simulink model "ARDroneHover_AMOSTROU"  (R2017b)
settings: Solver=ode1  StartTime=0.0  StopTime=inf  FixedStep=sampleTime  RelTol=1e-3  EnableMultiTasking=on
values from neighbouring files (symbols this model uses):
  sampleTime = 1/200    (= 0.005)    [setupWPTracking.m]
undefined symbols (not defined in the file or in its folder): Standard_Devices, UDP_Protocol
libraries: sldrtlib x3, ARBlocks x2
(part 1 of 2)
CloseFcn:
  | rtwprivate ssgencode ModelCloseRequest Good_NL_model
settings Model: SimulationMode=external  ExtModeTrigDuration=100000  Creator=Paul  LastModifiedBy=PauloOliveira
settings DataIOCC: LimitDataPoints=on  SaveFormat=Array  SignalLoggingSaveFormat=ModelDataLogs  TimeSaveName=time
settings OptimizationCC: ExpressionDepthLimit=2147483647  InitFltsAndDblsToZero=on
settings DebuggingCC: UnderspecifiedInitializationDetection=Classic  MergeDetectMultiDrivingBlocksExec=none  SolverPrmCheckMsg=warning  FcnCallInpInsideContextMsg=warning  StateNameClashWarn=warning  SFUnexpectedBacktrackingDiag=warning  SFNoUnconditionalDefaultTransitionDiag=warning  SFExecutionAtInitializationDiag=none
settings HardwareCC: ProdBitPerLong=64  ProdHWDeviceType=Intel->x86-64 (Mac OS X)
settings ModelReferenceCC: PropagateSignalLabelsOutOfModel=off
settings RTWCC: SystemTargetFile=sldrt.tlc  TemplateMakefile=sldrt.tmf  Description=Simulink Desktop Real-Time  RTWCompilerOptimization=on
settings CodeAppCC: MaxIdLength=95  StateflowObjectComments=on
settings SimulinkDesktopRealTimeCC: TargetPreCompLibLocation=/Applications/MATLAB_R2017b.app/toolbox/sldrt/lib/maci64  TargetLangStandard=C89/C90 (ANSI)  SupportVariableSizeSignals=off
settings ConfigComp: CovMetricSettings=dw  CovHtmlReporting=on  CovSaveCumulativeToWorkspaceVar=on  CovSaveSingleToWorkspaceVar=on  CovExternalEMLEnable=off

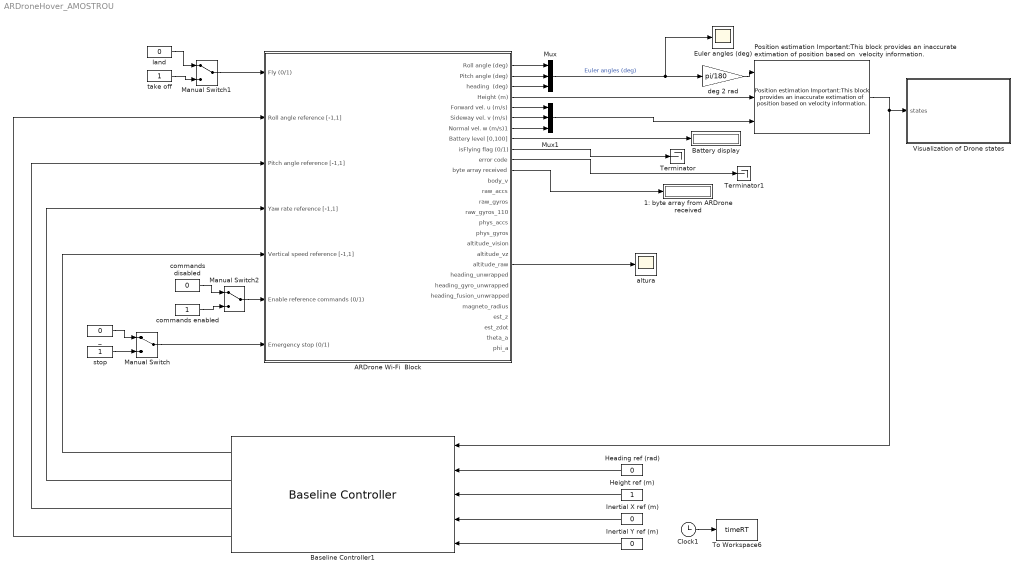
== system ARDroneHover_AMOSTROU ==
  "1: byte array from ARDrone received " : Display
  ARDrone Wi-Fi  Block : Subsystem  AncestorBlock="ARBlocks/ARDrone Wi-Fi  Block"
  Baseline Controller1 : ARBlocks/Baseline Controller
  Battery display : Display
  Clock1 : Clock
  Euler angles (deg) : Scope
  Heading ref (rad) : Constant  Value=0
  Height ref (m) : Constant
  Inertial X ref (m) : Constant  Value=0
  Inertial Y ref (m) : Constant  Value=0
  Manual Switch : ManualSwitch
  Manual Switch1 : ManualSwitch
  Manual Switch2 : ManualSwitch
  Mux : Mux  Inputs=3
  Mux1 : Mux  Inputs=3
  "Position estimation Important:This block provides an inaccurate extimation of position based on  velocity information. " : ARBlocks/Position estimation Important:This block provides an  inaccurate extimation of position  based on  velocity information. 
  Terminator : Terminator
  Terminator1 : Terminator
  To Workspace6 : ToWorkspace  VariableName=timeRT  SampleTime=sampleTime
  Visualization of Drone states : Subsystem
  _ : Constant  Value=0
  altura : Scope
  commands disabled : Constant  Value=0
  commands enabled : Constant
  deg 2 rad : Gain  Gain=pi/180
  land : Constant  Value=0
  stop : Constant
  take off : Constant
  wires:
  _/1 -> Manual Switch/1
  stop/1 -> Manual Switch/2
  land/1 -> Manual Switch1/1
  take off/1 -> Manual Switch1/2
  commands disabled/1 -> Manual Switch2/1
  commands enabled/1 -> Manual Switch2/2
  Manual Switch1/1 -> ARDrone Wi-Fi  Block/1(Fly (0/1))
  Manual Switch2/1 -> ARDrone Wi-Fi  Block/6(Enable reference commands (0/1))
  Manual Switch/1 -> ARDrone Wi-Fi  Block/7(Emergency stop (0/1))
  ARDrone Wi-Fi  Block/1(Roll angle (deg)) -> Mux/1
  ARDrone Wi-Fi  Block/2(Pitch angle (deg)) -> Mux/2
  ARDrone Wi-Fi  Block/5(Forward vel. u (m/s)) -> Mux1/1
  ARDrone Wi-Fi  Block/6(Sideway vel. v (m/s)) -> Mux1/2
  ARDrone Wi-Fi  Block/7(Normal vel. w (m/s)1) -> Mux1/3
  Mux/1 -> Euler angles (deg)/1, deg 2 rad/1  "Euler angles (deg)"
  ARDrone Wi-Fi  Block/8(Battery level [0,100]) -> Battery display/1
  Baseline Controller1/1 -> ARDrone Wi-Fi  Block/5(Vertical speed reference [-1,1])
  Baseline Controller1/3 -> ARDrone Wi-Fi  Block/3(Pitch angle reference [-1,1])
  "Position estimation Important:This block provides an inaccurate extimation of position based on  velocity information. "/1 -> Visualization of Drone states/1(states), Baseline Controller1/1
  deg 2 rad/1 -> "Position estimation Important:This block provides an inaccurate extimation of position based on  velocity information. "/1
  ARDrone Wi-Fi  Block/4(Height (m)) -> "Position estimation Important:This block provides an inaccurate extimation of position based on  velocity information. "/2
  Mux1/1 -> "Position estimation Important:This block provides an inaccurate extimation of position based on  velocity information. "/3
  Baseline Controller1/4 -> ARDrone Wi-Fi  Block/2(Roll angle reference [-1,1])
  ARDrone Wi-Fi  Block/3(heading  (deg)) -> Mux/3
  ARDrone Wi-Fi  Block/9(isFlying flag (0/1)) -> Terminator/1
  ARDrone Wi-Fi  Block/10(error code) -> Terminator1/1
  ARDrone Wi-Fi  Block/11(byte array received) -> "1: byte array from ARDrone received "/1
  Baseline Controller1/2 -> ARDrone Wi-Fi  Block/4(Yaw rate reference [-1,1])
  Clock1/1 -> To Workspace6/1
  Height ref (m)/1 -> Baseline Controller1/3
  Inertial X ref (m)/1 -> Baseline Controller1/4
  Inertial Y ref (m)/1 -> Baseline Controller1/5
  Heading ref (rad)/1 -> Baseline Controller1/2
  ARDrone Wi-Fi  Block/20(altitude_raw) -> altura/1

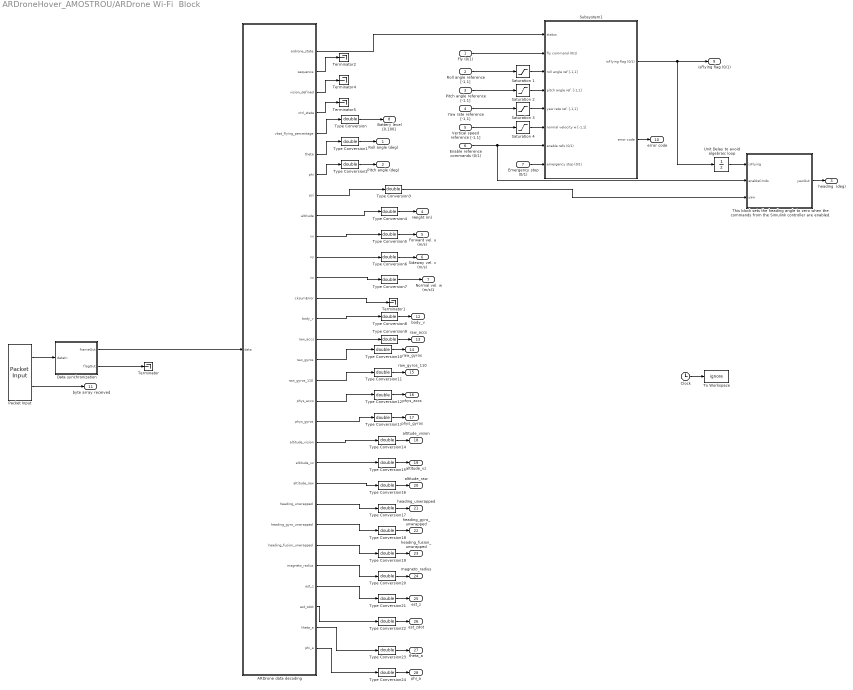
== system ARDroneHover_AMOSTROU/ARDrone Wi-Fi  Block ==
  Fly (0/1) : Inport
  Roll angle reference [-1,1] : Inport  Port=2
  Pitch angle reference [-1,1] : Inport  Port=3
  Yaw rate reference [-1,1] : Inport  Port=4
  Vertical speed reference [-1,1] : Inport  Port=5
  Enable reference commands (0/1) : Inport  Port=6
  Emergency stop (0/1) : Inport  Port=7
  ARDrone data decoding : MATLAB Function  TreatAsAtomicUnit=on
  Clock : Clock
      settings: Decimation=100
  "Data synchronization " : MATLAB Function  TreatAsAtomicUnit=on
  Packet Input : sldrtlib/Packet Input  SampleTime=sampleTime  MaxMissedTicks=100  ShowMissedTicks=off  YieldWhenWaiting=off  DrvName=Standard_Devices/UDP_Protocol  DrvAddress=5554  DrvOptions=[3232235777 5554]  PacketSize=2190  DataTypes='2190*uint8'  ShowReady=on  ShowError=off  PacketID=1  ByteOrder=1  ShowTimestamp=off
      settings: AttributesFormatString=UDP Protocol [5554]  SourceProductName=Simulink Desktop Real-Time
  Saturation {1..4} (4 alike) : Saturate  UpperLimit=1  LowerLimit=-1
  Subsystem1 : Subsystem
  Terminator{,1..2,4..5} (5 alike) : Terminator
  "This block sets the heading angle to zero when the commands from the Simulink controller are enabled. " : MATLAB Function  TreatAsAtomicUnit=on
  To Workspace : ToWorkspace  VariableName=ignore  SaveFormat=Timeseries  SampleTime=-1
  Type Conversion{,1..24} (25 alike) : DataTypeConversion  OutDataTypeStr=double
  Unit Delay to avoid algebraic loop : UnitDelay  SampleTime=-1
  Roll angle (deg) : Outport
  Pitch angle (deg) : Outport  Port=2
  heading  (deg) : Outport  Port=3
  Height (m) : Outport  Port=4
  Forward vel. u (m/s) : Outport  Port=5
  Sideway vel. v (m/s) : Outport  Port=6
  Normal vel. w (m/s)1 : Outport  Port=7
  Battery level [0,100] : Outport  Port=8
  isFlying flag (0/1) : Outport  Port=9
  error code : Outport  Port=10
  byte array received : Outport  Port=11
  body_v : Outport  Port=12
  raw_accs : Outport  Port=13
  raw_gyros : Outport  Port=14
  raw_gyros_110 : Outport  Port=15
  phys_accs : Outport  Port=16
  phys_gyros : Outport  Port=17
  altitude_vision : Outport  Port=18
  altitude_vz : Outport  Port=19
  altitude_raw : Outport  Port=20
  heading_unwrapped : Outport  Port=21
  heading_gyro_unwrapped : Outport  Port=22
  heading_fusion_unwrapped : Outport  Port=23
  magneto_radius : Outport  Port=24
  est_z : Outport  Port=25
  est_zdot : Outport  Port=26
  theta_a : Outport  Port=27
  phi_a : Outport  Port=28
  wires:
  Packet Input/1 -> "Data synchronization "/1(dataIn)
  "Data synchronization "/1(frameOut) -> ARDrone data decoding/1(data)
  Packet Input/2 -> byte array received/1
  ARDrone data decoding/1(ardrone_state) -> Subsystem1/1(status)
  Roll angle reference [-1,1]/1 -> Saturation 1/1
  Pitch angle reference [-1,1]/1 -> Saturation 2/1
  Yaw rate reference [-1,1]/1 -> Saturation 3/1
  Vertical speed reference [-1,1]/1 -> Saturation 4/1
  Enable reference commands (0/1)/1 -> "This block sets the heading angle to zero when the commands from the Simulink controller are enabled. "/2(enableCmds), Subsystem1/7(enable refs (0/1))
  Emergency stop (0/1)/1 -> Subsystem1/8(emergency stop (0/1))
  Subsystem1/1(isFlying flag (0/1)) -> isFlying flag (0/1)/1, Unit Delay to avoid algebraic loop/1
  Subsystem1/2(error code) -> error code/1
  ARDrone data decoding/13(cksumError) -> Terminator1/1
  Type Conversion/1 -> Battery level [0,100]/1
  Type Conversion1/1 -> Roll angle (deg)/1
  Type Conversion2/1 -> Pitch angle (deg)/1
  Type Conversion4/1 -> Height (m)/1
  Type Conversion5/1 -> Forward vel. u (m/s)/1
  Type Conversion6/1 -> Sideway vel. v (m/s)/1
  Type Conversion7/1 -> Normal vel. w (m/s)1/1
  Type Conversion3/1 -> "This block sets the heading angle to zero when the commands from the Simulink controller are enabled. "/3(yaw)
  "This block sets the heading angle to zero when the commands from the Simulink controller are enabled. "/1(yawOut) -> heading  (deg)/1
  Fly (0/1)/1 -> Subsystem1/2(fly command (0/1))
  Saturation 1/1 -> Subsystem1/3(roll angle ref [-1,1])
  Saturation 2/1 -> Subsystem1/4(pitch angle ref. [-1,1])
  Saturation 3/1 -> Subsystem1/5(yaw rate ref. [-1,1])
  Saturation 4/1 -> Subsystem1/6(normal velocity w [-1,1])
  "Data synchronization "/2(flagOut) -> Terminator/1
  Unit Delay to avoid algebraic loop/1 -> "This block sets the heading angle to zero when the commands from the Simulink controller are enabled. "/1(isFlying)
  Clock/1 -> To Workspace/1
  ARDrone data decoding/12(vz) -> Type Conversion7/1
  ARDrone data decoding/11(vy) -> Type Conversion6/1
  ARDrone data decoding/10(vx) -> Type Conversion5/1
  ARDrone data decoding/9(altitude) -> Type Conversion4/1
  ARDrone data decoding/8(psi) -> Type Conversion3/1
  ARDrone data decoding/7(phi) -> Type Conversion2/1
  ARDrone data decoding/6(theta) -> Type Conversion1/1
  ARDrone data decoding/5(vbat_flying_percentage) -> Type Conversion/1
  ARDrone data decoding/2(sequence) -> Terminator2/1
  ARDrone data decoding/3(vision_defined) -> Terminator4/1
  ARDrone data decoding/4(ctrl_state) -> Terminator5/1
  Type Conversion8/1 -> body_v/1
  Type Conversion9/1 -> raw_accs/1
  Type Conversion10/1 -> raw_gyros/1
  Type Conversion11/1 -> raw_gyros_110/1
  Type Conversion12/1 -> phys_accs/1
  Type Conversion13/1 -> phys_gyros/1
  ARDrone data decoding/19(phys_gyros) -> Type Conversion13/1
  Type Conversion14/1 -> altitude_vision/1
  Type Conversion15/1 -> altitude_vz/1
  Type Conversion16/1 -> altitude_raw/1
  Type Conversion17/1 -> heading_unwrapped/1
  Type Conversion18/1 -> heading_gyro_unwrapped/1
  Type Conversion19/1 -> heading_fusion_unwrapped/1
  Type Conversion20/1 -> magneto_radius/1
  Type Conversion21/1 -> est_z/1
  Type Conversion22/1 -> est_zdot/1
  ARDrone data decoding/28(est_zdot) -> Type Conversion22/1
  Type Conversion23/1 -> theta_a/1
  Type Conversion24/1 -> phi_a/1
  ARDrone data decoding/29(theta_a) -> Type Conversion23/1
  ARDrone data decoding/30(phi_a) -> Type Conversion24/1
  ARDrone data decoding/14(body_v) -> Type Conversion8/1
  ARDrone data decoding/15(raw_accs) -> Type Conversion9/1
  ARDrone data decoding/16(raw_gyros) -> Type Conversion10/1
  ARDrone data decoding/17(raw_gyros_110) -> Type Conversion11/1
  ARDrone data decoding/18(phys_accs) -> Type Conversion12/1
  ARDrone data decoding/20(altitude_vision) -> Type Conversion14/1
  ARDrone data decoding/21(altitude_vz) -> Type Conversion15/1
  ARDrone data decoding/22(altitude_raw) -> Type Conversion16/1
  ARDrone data decoding/23(heading_unwrapped) -> Type Conversion17/1
  ARDrone data decoding/24(heading_gyro_unwrapped) -> Type Conversion18/1
  ARDrone data decoding/25(heading_fusion_unwrapped) -> Type Conversion19/1
  ARDrone data decoding/26(magneto_radius) -> Type Conversion20/1
  ARDrone data decoding/27(est_z) -> Type Conversion21/1

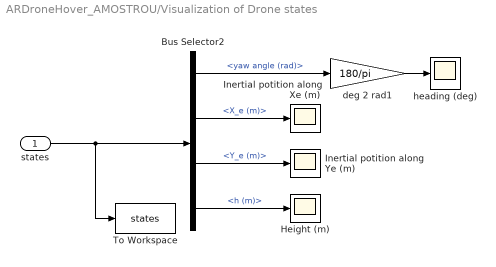
== system ARDroneHover_AMOSTROU/Visualization of Drone states ==
  states : Inport
  Bus Selector2 : BusSelector  OutputSignals=yaw angle (rad),X_e (m),Y_e (m),h (m)
  Height (m) : Scope
  Inertial potition along Xe (m) : Scope
  Inertial potition along Ye (m) : Scope
  To Workspace : ToWorkspace  VariableName=states  SaveFormat=Structure With Time  SampleTime=-1
  deg 2 rad1 : Gain  Gain=180/pi
  heading (deg) : Scope
  wires:
  states/1 -> To Workspace/1, Bus Selector2/1
  Bus Selector2/1 -> deg 2 rad1/1  "<yaw angle (rad)>"
  Bus Selector2/2 -> Inertial potition along Xe (m)/1  "<X_e (m)>"
  Bus Selector2/3 -> Inertial potition along Ye (m)/1  "<Y_e (m)>"
  Bus Selector2/4 -> Height (m)/1  "<h (m)>"
  deg 2 rad1/1 -> heading (deg)/1

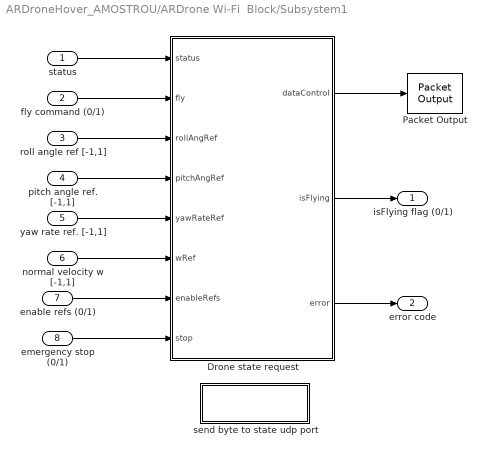
== system ARDroneHover_AMOSTROU/ARDrone Wi-Fi  Block/Subsystem1 ==
  status : Inport
  fly command (0/1) : Inport  Port=2
  roll angle ref [-1,1] : Inport  Port=3
  pitch angle ref. [-1,1] : Inport  Port=4
  yaw rate ref. [-1,1] : Inport  Port=5
  normal velocity w [-1,1] : Inport  Port=6
  enable refs (0/1) : Inport  Port=7
  emergency stop (0/1) : Inport  Port=8
  Drone state request : MATLAB Function  TreatAsAtomicUnit=on  SystemSampleTime=sampleTime
  Packet Output : sldrtlib/Packet Output  SampleTime=-1  MaxMissedTicks=100  ShowMissedTicks=off  YieldWhenWaiting=off  DrvName=Standard_Devices/UDP_Protocol  DrvAddress=5556  DrvOptions=[3232235777 5556]  PacketSize=150  DataTypes='150*uint8'  ShowReady=off  ShowError=off  PacketID=1  ByteOrder=1  InitialValue=[]  FinalValue=[]
      settings: AttributesFormatString=UDP Protocol [5556]  SourceProductName=Simulink Desktop Real-Time
  "send byte to state udp port " : Subsystem
  isFlying flag (0/1) : Outport
  error code : Outport  Port=2
  wires:
  fly command (0/1)/1 -> Drone state request/2(fly)
  pitch angle ref. [-1,1]/1 -> Drone state request/4(pitchAngRef)
  status/1 -> Drone state request/1(status)
  Drone state request/1(dataControl) -> Packet Output/1
  Drone state request/2(isFlying) -> isFlying flag (0/1)/1
  roll angle ref [-1,1]/1 -> Drone state request/3(rollAngRef)
  yaw rate ref. [-1,1]/1 -> Drone state request/5(yawRateRef)
  normal velocity w [-1,1]/1 -> Drone state request/6(wRef)
  enable refs (0/1)/1 -> Drone state request/7(enableRefs)
  emergency stop (0/1)/1 -> Drone state request/8(stop)
  Drone state request/3(error) -> error code/1

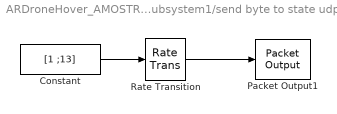
== system ARDroneHover_AMOSTROU/ARDrone Wi-Fi  Block/Subsystem1/send byte to state udp port  ==
  Constant : Constant  Value=[1 ;13]  OutDataTypeStr=uint8
  Packet Output1 : sldrtlib/Packet Output  SampleTime=sampleTime*10  MaxMissedTicks=100  ShowMissedTicks=off  YieldWhenWaiting=off  DrvName=Standard_Devices/UDP_Protocol  DrvAddress=5554  DrvOptions=[3232235777 5554]  PacketSize=2  DataTypes='2*uint8'  ShowReady=off  ShowError=off  PacketID=1  ByteOrder=1  InitialValue=[]  FinalValue=[]
      settings: AttributesFormatString=UDP Protocol [5554]  SourceProductName=Simulink Desktop Real-Time
  Rate Transition : RateTransition  OutPortSampleTime=sampleTime*10
  wires:
  Constant/1 -> Rate Transition/1
  Rate Transition/1 -> Packet Output1/1

== matlab function ARDroneHover_AMOSTROU/ARDrone Wi-Fi  Block/ARDrone data decoding ==
  data: ardrone_state output; sequence output; vision_defined output; data input; ctrl_state output; vbat_flying_percentage output; theta output; phi output; psi output; altitude output; vx output; vy output; vz output; cksumError output; body_v output; raw_accs output; raw_gyros output; raw_gyros_110 output; phys_accs output; phys_gyros output; altitude_vision output; altitude_vz output; altitude_raw output; heading_unwrapped output; heading_gyro_unwrapped output; heading_fusion_unwrapped output; magneto_radius output; est_z output; est_zdot output; theta_a output; phi_a output
function [ ardrone_state, sequence, vision_defined, ctrl_state, vbat_flying_percentage, theta, phi, psi, altitude, vx, vy, vz , cksumError , body_v,raw_accs,raw_gyros,raw_gyros_110,phys_accs,phys_gyros,altitude_vision,altitude_vz,altitude_raw,heading_unwrapped,heading_gyro_unwrapped,heading_fusion_unwrapped,magneto_radius,est_z,est_zdot,theta_a,phi_a]= fcn(data)
%#codegen

%initialie arrays
raw_accs=zeros(3,1);
raw_gyros=zeros(3,1);
raw_gyros_110=zeros(2,1);
phys_accs=zeros(3,1);
phys_gyros=zeros(3,1);
offsets_g=zeros(3,1);
obs_x=zeros(3,1);
est_vb=zeros(2,1);
of_dx=zeros(5,1);
of_dy=zeros(5,1);
body_v=zeros(3,1);
time_custom=zeros(20,1);
locked=zeros(30,1);
point=zeros(30,2);
type=zeros(4,1);
xc=zeros(4,1);
yc=zeros(4,1);
width=zeros(4,1);
height=zeros(4,1);
dist=zeros(4,1);
orientation_angle=zeros(4,1);
rotation=zeros(3,3,4);
translation=zeros(3,1,4);
camera_source=zeros(4,1);
data_frame=zeros(32,1);
magneto_raw=zeros(3,1);
magneto_rectified=zeros(3,1);
magneto_offset=zeros(3,1);

% Checksum array. cksum(1) contains the computed checksum, cksum(2)
% contains the checksum sent by the ARDrone. 
cksum = [0 0 ]; 

% Previous value of height 
persistent hPrev ; 
% Previous data packet
persistent dataPrev ; 

% Initialization of persistent variables
if isempty(hPrev)
    hPrev=0 ; 
end

if isempty(dataPrev)
    dataPrev = uint8(zeros(2186,1)) ;
end

% Computing checksum
cksum(1) =  sum(double(data(1:end-8))) +442; 
% Checksum given by the drone
cksum(2) = double(data(end-3)) + double(data(end-2))*256 +  double(data(end-1))*256^2 + double(data(end))*256^3 ; 
% Checksum error
cksumError = abs(cksum(1)-cksum(2));
%% Change the following if statement to ensure that the data checksum is valid 
%if (data(15) == 148 && cksumError==0 )
if (data(15) == 148  )
    dataPrev = data; 
else
    data = dataPrev; 
end

% Converting bytes to drone information

% header data
ardrone_state = getDroneState(data(1:4));
sequence = decode_32bit(data(5:8),1);
vision_defined = data(9);

% demo data
ctrl_state = decode_32bit(data(17:20),1);
vbat_flying_percentage = decode_32bit(data(21:24),1); % unit: deg
theta = decode_32bit(data(25:28),0)/1000; % unit: deg
phi = decode_32bit(data(29:32),0)/1000; % unit: deg
psi = decode_32bit(data(33:36),0)/1000; % unit: deg
altitude = decode_32bit(data(37:40),1)/1000; % unit: deg
vx = decode_32bit(data(41:44),0)/1000; % unit: m/s
vy = decode_32bit(data(45:48),0)/1000; % unit: m/s
vz = decode_32bit(data(49:52),0)/1000; % unit: m/s
detection_camera_type = decode_32bit(data(109:112),1);

%altitude = decode_32bit(data(113:116),1)/1000;

% time !!!!CHECK UNITS!!!!
time = decode_32bit(data(165:168),1);

% raw data
raw_accs(1) = decode_16bit(data(173:174),0);
raw_accs(2) = decode_16bit(data(175:176),0);
raw_accs(3) = decode_16bit(data(177:178),0);
raw_gyros(1) = decode_16bit(data(179:180),1);
raw_gyros(2) = decode_16bit(data(181:182),1);
raw_gyros(3) = decode_16bit(data(183:184),1);
raw_gyros_110(1) = decode_16bit(data(185:186),1);
raw_gyros_110(2) = decode_16bit(data(187:188),1);
vbat_raw = decode_32bit(data(189:192),0);
us_debut_echo = decode_16bit(data(193:194),0);
us_fin_echo = decode_16bit(data(195:196),0);
us_association_echo = decode_16bit(data(197:198),0);
us_distance_echo = decode_16bit(data(199:200),0);
us_courbe_temps = decode_16bit(data(201:202),0);
us_courbe_valeur = decode_16bit(data(203:204),0);
us_courbe_ref = decode_16bit(data(205:206),0);
flag_echo_ini = decode_16bit(data(207:208),0);
nb_echo = decode_16bit(data(209:210),0);
sum_echo = decode_32bit(data(211:214),1);
alt_temp_raw = decode_32bit(data(215:218),2);
gradient = decode_16bit(data(219:220),1);

% physycal measures
accs_temp = decode_32bit(data(225:228),0);
gyro_temp = decode_16bit(data(229:230),0);
phys_accs(1) = decode_32bit(data(231:234),0);
phys_accs(2) = decode_32bit(data(235:238),0);
phys_accs(3) = decode_32bit(data(239:242),0);
phys_gyros(1) = decode_32bit(data(243:246),0);
phys_gyros(2) = decode_32bit(data(247:250),0);
phys_gyros(3) = decode_32bit(data(251:254),0);
alim3V3 = decode_32bit(data(255:258),1);
vrefEpson = decode_32bit(data(259:262),1);
vrefIDG = decode_32bit(data(263:266),1);

% gyros offsets
offsets_g(1) = decode_32bit(data(271:274),0);
offsets_g(2) = decode_32bit(data(275:278),0);
offsets_g(3) = decode_32bit(data(279:282),0);

% euler angles
theta_a = decode_32bit(data(287:290),0);
phi_a = decode_32bit(data(291:294),0);

% referenes
ref_theta = decode_32bit(data(299:302),2);
ref_phi = decode_32bit(data(303:306),2);
ref_theta_I = decode_32bit(data(307:310),2);
ref_phi_I = decode_32bit(data(311:314),2);
ref_pitch = decode_32bit(data(315:318),2);
ref_roll = decode_32bit(data(319:322),2);
ref_yaw = decode_32bit(data(323:326),2);
ref_psi = decode_32bit(data(327:330),2);
vx_ref = decode_32bit(data(331:334),0);
vy_ref = decode_32bit(data(335:338),0);
theta_mod = decode_32bit(data(339:342),0);
phi_mod = decode_32bit(data(343:346),0);
k_v_x = decode_32bit(data(347:350),0);
k_v_y = decode_32bit(data(351:354),0);
k_mode = decode_32bit(data(355:358),1);
ui_time = decode_32bit(data(359:362),0);
ui_theta = decode_32bit(data(363:366),0);
ui_phi = decode_32bit(data(367:370),0);
ui_psi = decode_32bit(data(371:374),0);
ui_psi_accuracy = decode_32bit(data(375:378),0);
ui_seq = decode_32bit(data(379:382),2);

% trims
angular_rates_trim_r = decode_32bit(data(387:390),0);
euler_angles_trim_theta = decode_32bit(data(391:394),0);
euler_angles_trim_phi = decode_32bit(data(395:398),0);

% rc_refereces
rc_ref_pitch = decode_32bit(data(403:406),2);
rc_ref_roll = decode_32bit(data(407:410),2);
rc_ref_yaw = decode_32bit(data(411:414),2);
rc_ref_gaz = decode_32bit(data(415:418),2);
rc_ref_ag = decode_32bit(data(419:422),2);

% pwm
motor1 = data(427);
motor2 = data(428);
motor3 = data(429);
motor4 = data(430);
sat_motor1 = data(431);
sat_motor2 = data(432);
sat_motor3 = data(433);
sat_motor4 = data(434);
gaz_feed_forward = decode_32bit(data(435:438),0);
gaz_altitude = decode_32bit(data(439:442),0);
altitude_integral = decode_32bit(data(443:446),0);
vz_ref = decode_32bit(data(447:450),0);
u_pitch = decode_32bit(data(451:454),2);
u_roll = decode_32bit(data(455:458),2);
u_yaw = decode_32bit(data(459:462),2);
yaw_u_I = decode_32bit(data(463:466),0);
u_pitch_planif = decode_32bit(data(467:470),2);
u_roll_planif = decode_32bit(data(471:474),2);
u_yaw_planif = decode_32bit(data(475:478),2);
u_gaz_planif = decode_32bit(data(479:482),0);
current_motor1 = decode_16bit(data(483:484),0);
current_motor2 = decode_16bit(data(485:486),0);
current_motor3 = decode_16bit(data(487:488),0);
current_motor4 = decode_16bit(data(489:490),0);
altitude_prop = decode_32bit(data(491:494),0);
altitude_der = decode_32bit(data(495:498),0);

% altitude
altitude_vision = decode_32bit(data(519:522),2);
altitude_vz = decode_32bit(data(523:526),0);
altitude_ref = decode_32bit(data(527:530),2);
altitude_raw = decode_32bit(data(531:534),2);
obs_accZ = decode_32bit(data(535:538),0);
obs_alt = decode_32bit(data(539:542),0);
obs_x(1) = decode_32bit(data(543:546),0);
obs_x(2) = decode_32bit(data(547:550),0);
obs_x(3) = decode_32bit(data(551:554),0);
obs_state = decode_32bit(data(555:558),1);
est_vb(1) = decode_32bit(data(559:562),0);
est_vb(2) = decode_32bit(data(563:566),0);
est_state = decode_32bit(data(567:570),1);

% vision_raw
vision_tx_raw = decode_32bit(data(575:578),0);
vision_ty_raw = decode_32bit(data(579:582),0);
vision_tz_raw = decode_32bit(data(583:586),0);

% vision_of
of_dx(1) = decode_32bit(data(591:594),0);
of_dx(2) = decode_32bit(data(595:598),0);
of_dx(3) = decode_32bit(data(599:602),0);
of_dx(4) = decode_32bit(data(603:606),0);
of_dx(5) = decode_32bit(data(607:610),0);
of_dy(1) = decode_32bit(data(611:614),0);
of_dy(2) = decode_32bit(data(615:618),0);
of_dy(3) = decode_32bit(data(619:622),0);
of_dy(4) = decode_32bit(data(623:626),0);
of_dy(5) = decode_32bit(data(627:630),0);

% vision
vision_state = decode_32bit(data(635:638),1);
vision_misc = decode_32bit(data(639:642),2);
vision_phi_trim = decode_32bit(data(643:646),0);
vision_phi_ref_prop = decode_32bit(data(647:650),0);
vision_theta_trim = decode_32bit(data(651:654),0);
vision_theta_ref_prop = decode_32bit(data(655:658),0);
new_raw_picture = decode_32bit(data(659:662),2);
theta_capture = decode_32bit(data(663:666),0);
phi_capture = decode_32bit(data(667:670),0);
psi_capture = decode_32bit(data(671:674),0);
altitude_capture = decode_32bit(data(675:678),2);
time_capture = decode_32bit(data(679:682),1);
body_v(1) = decode_32bit(data(683:686),0);
body_v(2) = decode_32bit(data(687:690),0);
body_v(3) = decode_32bit(data(691:694),0);
delta_phi = decode_32bit(data(695:698),0);
delta_theta = decode_32bit(data(699:702),0);
delta_psi = decode_32bit(data(703:706),0);
gold_defined = decode_32bit(data(707:710),1);
gold_reset = decode_32bit(data(711:714),1);
gold_x = decode_32bit(data(715:718),0);
gold_y = decode_32bit(data(719:722),0);

% vision perf
time_szo = decode_32bit(data(727:730),0);
time_corners = decode_32bit(data(731:734),0);
time_compute = decode_32bit(data(725:738),0);
time_tracking = decode_32bit(data(739:742),0);
time_trans = decode_32bit(data(743:746),0);
time_update = decode_32bit(data(747:750),0);
time_custom(1) = decode_32bit(data(751:754),0);
time_custom(2) = decode_32bit(data(755:758),0);
time_custom(3) = decode_32bit(data(759:762),0);
time_custom(4) = decode_32bit(data(763:766),0);
time_custom(5) = decode_32bit(data(767:770),0);
time_custom(6) = decode_32bit(data(771:774),0);
time_custom(7) = decode_32bit(data(775:778),0);
time_custom(8) = decode_32bit(data(779:782),0);
time_custom(9) = decode_32bit(data(783:786),0);
time_custom(10) = decode_32bit(data(787:790),0);
time_custom(11) = decode_32bit(data(791:794),0);
time_custom(12) = decode_32bit(data(795:798),0);
time_custom(13) = decode_32bit(data(799:802),0);
time_custom(14) = decode_32bit(data(803:806),0);
time_custom(15) = decode_32bit(data(807:810),0);
time_custom(16) = decode_32bit(data(811:814),0);
time_custom(17) = decode_32bit(data(815:818),0);
time_custom(18) = decode_32bit(data(819:822),0);
time_custom(19) = decode_32bit(data(823:826),0);
time_custom(20) = decode_32bit(data(827:830),0);

% trackers send
locked(1) = decode_32bit(data(835:838),2);
locked(2) = decode_32bit(data(839:842),2);
locked(3) = decode_32bit(data(843:846),2);
locked(4) = decode_32bit(data(847:850),2);
locked(5) = decode_32bit(data(851:854),2);
locked(6) = decode_32bit(data(855:858),2);
locked(7) = decode_32bit(data(859:862),2);
locked(8) = decode_32bit(data(863:866),2);
locked(9) = decode_32bit(data(867:870),2);
locked(10) = decode_32bit(data(871:874),2);
locked(11) = decode_32bit(data(875:878),2);
locked(12) = decode_32bit(data(879:882),2);
locked(13) = decode_32bit(data(883:886),2);
locked(14) = decode_32bit(data(887:890),2);
locked(15) = decode_32bit(data(891:894),2);
locked(16) = decode_32bit(data(895:898),2);
locked(17) = decode_32bit(data(899:902),2);
locked(18) = decode_32bit(data(903:906),2);
locked(19) = decode_32bit(data(907:910),2);
locked(20) = decode_32bit(data(911:914),2);
locked(21) = decode_32bit(data(915:918),2);
locked(22) = decode_32bit(data(919:922),2);
locked(23) = decode_32bit(data(923:926),2);
locked(24) = decode_32bit(data(927:930),2);
locked(25) = decode_32bit(data(931:934),2);
locked(26) = decode_32bit(data(935:938),2);
locked(27) = decode_32bit(data(939:942),2);
locked(28) = decode_32bit(data(943:946),2);
locked(29) = decode_32bit(data(947:950),2);
locked(30) = decode_32bit(data(951:954),2);
point(1,1) = decode_32bit(data(955:958),0);
point(1,2) = decode_32bit(data(959:962),0);
point(2,1) = decode_32bit(data(963:966),0);
point(2,2) = decode_32bit(data(967:970),0);
point(3,1) = decode_32bit(data(971:974),0);
point(3,2) = decode_32bit(data(975:978),0);
point(4,1) = decode_32bit(data(979:982),0);
point(4,2) = decode_32bit(data(983:986),0);
point(5,1) = decode_32bit(data(987:990),0);
point(5,2) = decode_32bit(data(991:994),0);
point(6,1) = decode_32bit(data(995:998),0);
point(6,2) = decode_32bit(data(999:1002),0);
point(7,1) = decode_32bit(data(1003:1006),0);
point(7,2) = decode_32bit(data(1007:1010),0);
point(8,1) = decode_32bit(data(1011:1014),0);
point(8,2) = decode_32bit(data(1015:1018),0);
point(9,1) = decode_32bit(data(1019:1022),0);
point(9,2) = decode_32bit(data(1023:1026),0);
point(10,1) = decode_32bit(data(1027:1030),0);
point(10,2) = decode_32bit(data(1031:1034),0);
point(11,1) = decode_32bit(data(1035:1038),0);
point(11,2) = decode_32bit(data(1039:1042),0);
point(12,1) = decode_32bit(data(1043:1046),0);
point(12,2) = decode_32bit(data(1047:1050),0);
point(13,1) = decode_32bit(data(1051:1054),0);
point(13,2) = decode_32bit(data(1055:1058),0);
point(14,1) = decode_32bit(data(1059:1062),0);
point(14,2) = decode_32bit(data(1063:1066),0);
point(15,1) = decode_32bit(data(1067:1070),0);
point(15,2) = decode_32bit(data(1071:1074),0);
point(16,1) = decode_32bit(data(1075:1078),0);
point(16,2) = decode_32bit(data(1079:1082),0);
point(17,1) = decode_32bit(data(1083:1086),0);
point(17,2) = decode_32bit(data(1087:1090),0);
point(18,1) = decode_32bit(data(1091:1094),0);
point(18,2) = decode_32bit(data(1095:1098),0);
point(19,1) = decode_32bit(data(1099:1102),0);
point(19,2) = decode_32bit(data(1103:1106),0);
point(20,1) = decode_32bit(data(1107:1110),0);
point(20,2) = decode_32bit(data(1111:1114),0);
point(21,1) = decode_32bit(data(1115:1118),0);
point(21,2) = decode_32bit(data(1119:1122),0);
point(22,1) = decode_32bit(data(1123:1126),0);
point(22,2) = decode_32bit(data(1127:1130),0);
point(23,1) = decode_32bit(data(1131:1134),0);
point(23,2) = decode_32bit(data(1135:1138),0);
point(24,1) = decode_32bit(data(1139:1142),0);
point(24,2) = decode_32bit(data(1143:1146),0);
point(25,1) = decode_32bit(data(1147:1150),0);
point(25,2) = decode_32bit(data(1151:1154),0);
point(26,1) = decode_32bit(data(1155:1158),0);
point(26,2) = decode_32bit(data(1159:1162),0);
point(27,1) = decode_32bit(data(1163:1166),0);
point(27,2) = decode_32bit(data(1167:1170),0);
point(28,1) = decode_32bit(data(1171:1174),0);
point(28,2) = decode_32bit(data(1175:1178),0);
point(29,1) = decode_32bit(data(1179:1182),0);
point(29,2) = decode_32bit(data(1183:1186),0);
point(30,1) = decode_32bit(data(1187:1190),0);
point(30,2) = decode_32bit(data(1191:1194),0);

% vision detect
nb_detected = decode_32bit(data(1199:1202),1);
type(1) = decode_32bit(data(1203:1206),1);
type(2) = decode_32bit(data(1207:1210),1);
type(3) = decode_32bit(data(1211:1214),1);
type(4) = decode_32bit(data(1215:1218),1);
xc(1) = decode_32bit(data(1219:1222),1);
xc(2) = decode_32bit(data(1223:1226),1);
xc(3) = decode_32bit(data(1227:1230),1);
xc(4) = decode_32bit(data(1231:1234),1);
yc(1) = decode_32bit(data(1235:1238),1);
yc(2) = decode_32bit(data(1239:1242),1);
yc(3) = decode_32bit(data(1243:1246),1);
yc(4) = decode_32bit(data(1247:1250),1);
width(1) = decode_32bit(data(1251:1254),1);
width(2) = decode_32bit(data(1255:1258),1);
width(3) = decode_32bit(data(1259:1262),1);
width(4) = decode_32bit(data(1263:1266),1);
height(1) = decode_32bit(data(1267:1270),1);
height(2) = decode_32bit(data(1271:1274),1);
height(3) = decode_32bit(data(1275:1278),1);
height(4) = decode_32bit(data(1279:1282),1);
dist(1) = decode_32bit(data(1283:1286),1);
dist(2) = decode_32bit(data(1287:1290),1);
dist(3) = decode_32bit(data(1291:1294),1);
dist(4) = decode_32bit(data(1295:1298),1);
orientation_angle(1) = decode_32bit(data(1299:1302),0);
orientation_angle(2) = decode_32bit(data(1303:1306),0);
orientation_angle(3) = decode_32bit(data(1307:1310),0);
orientation_angle(4) = decode_32bit(data(131:1314),0);
rotation(1,1,1) = decode_32bit(data(1315:1318),0);
rotation(1,2,1) = decode_32bit(data(1319:1322),0);
rotation(1,3,1) = decode_32bit(data(1323:1326),0);
rotation(2,1,1) = decode_32bit(data(1327:1330),0);
rotation(2,2,1) = decode_32bit(data(1331:1334),0);
rotation(2,3,1) = decode_32bit(data(1335:1338),0);
rotation(3,1,1) = decode_32bit(data(1339:1342),0);
rotation(3,2,1) = decode_32bit(data(1343:1346),0);
rotation(3,3,1) = decode_32bit(data(1347:1350),0);
rotation(1,1,2) = decode_32bit(data(1351:1354),0);
rotation(1,2,2) = decode_32bit(data(1355:1358),0);
rotation(1,3,2) = decode_32bit(data(1359:1362),0);
rotation(2,1,2) = decode_32bit(data(1363:1366),0);
rotation(2,2,2) = decode_32bit(data(1367:1370),0);
rotation(2,3,2) = decode_32bit(data(1371:1374),0);
rotation(3,1,2) = decode_32bit(data(1375:1378),0);
rotation(3,2,2) = decode_32bit(data(1379:1382),0);
rotation(3,3,2) = decode_32bit(data(1383:1386),0);
rotation(1,1,3) = decode_32bit(data(1387:1390),0);
rotation(1,2,3) = decode_32bit(data(1391:1394),0);
rotation(1,3,3) = decode_32bit(data(1395:1398),0);
rotation(2,1,3) = decode_32bit(data(1399:1402),0);
rotation(2,2,3) = decode_32bit(data(1403:1406),0);
rotation(2,3,3) = decode_32bit(data(1407:1410),0);
rotation(3,1,3) = decode_32bit(data(1411:1414),0);
rotation(3,2,3) = decode_32bit(data(1415:1418),0);
rotation(3,3,3) = decode_32bit(data(1419:1422),0);
rotation(1,1,4) = decode_32bit(data(1423:1426),0);
rotation(1,2,4) = decode_32bit(data(1427:1430),0);
rotation(1,3,4) = decode_32bit(data(1431:1434),0);
rotation(2,1,4) = decode_32bit(data(1435:1438),0);
rotation(2,2,4) = decode_32bit(data(1439:1442),0);
rotation(2,3,4) = decode_32bit(data(1443:1446),0);
rotation(3,1,4) = decode_32bit(data(1447:1450),0);
rotation(3,2,4) = decode_32bit(data(1451:1454),0);
rotation(3,3,4) = decode_32bit(data(1455:1458),0);
translation(1,1,1) = decode_32bit(data(1459:1462),0);
translation(1,1,1) = decode_32bit(data(1463:1466),0);
translation(3,1,1) = decode_32bit(data(1467:1470),0);
translation(1,1,2) = decode_32bit(data(1471:1474),0);
translation(2,1,2) = decode_32bit(data(1475:1478),0);
translation(3,1,2) = decode_32bit(data(1479:1482),0);
translation(1,1,3) = decode_32bit(data(1483:1486),0);
translation(2,1,3) = decode_32bit(data(1487:1490),0);
translation(3,1,3) = decode_32bit(data(1491:1494),0);
translation(1,1,4) = decode_32bit(data(1495:1498),0);
translation(2,1,4) = decode_32bit(data(1499:1502),0);
translation(3,1,4) = decode_32bit(data(1503:1506),0);
camera_source(1) = decode_32bit(data(1507:1510),1);
camera_source(2) = decode_32bit(data(1511:1514),1);
camera_source(3) = decode_32bit(data(1515:1518),1);
camera_source(4) = decode_32bit(data(1519:1522),1);

% watchdog
watchdog = decode_32bit(data(1527:1530),2);

% adc data frame
version = decode_32bit(data(1535:1538),1);
data_frame(1) = data(1539);
data_frame(2) = data(1540);
data_frame(3) = data(1541);
data_frame(4) = data(1542);
data_frame(5) = data(1543);
data_frame(6) = data(1544);
data_frame(7) = data(1545);
data_frame(8) = data(1546);
data_frame(9) = data(1547);
data_frame(10) = data(1548);
data_frame(11) = data(1549);
data_frame(12) = data(1550);
data_frame(13) = data(1551);
data_frame(14) = data(1552);
data_frame(15) = data(1553);
data_frame(16) = data(1554);
data_frame(17) = data(1555);
data_frame(18) = data(1556);
data_frame(19) = data(1557);
data_frame(20) = data(1558);
data_frame(21) = data(1559);
data_frame(22) = data(1560);
data_frame(23) = data(1561);
data_frame(24) = data(1562);
data_frame(25) = data(1563);
data_frame(26) = data(1564);
data_frame(27) = data(1565);
data_frame(28) = data(1566);
data_frame(29) = data(1567);
data_frame(30) = data(1568);
data_frame(31) = data(1569);
data_frame(32) = data(1570);

% video stream
quant = data(1575);
frame_size = decode_32bit(data(1576:1579),1);
frame_number = decode_32bit(data(1580:1583),1);
atcmd_ref_seq = decode_32bit(data(1584:1587),1);
atcmd_mean_ref_gap = decode_32bit(data(1588:1591),1);
atcmd_var_ref_gap = decode_32bit(data(1592:1595),0);
atcmd_ref_quality = decode_32bit(data(1596:1599),1);
out_bitrate = decode_32bit(data(1600:1603),1);
desired_bitrate = decode_32bit(data(1604:1607),1);
data1 = decode_32bit(data(1608:1611),2);
data2 = decode_32bit(data(1612:1615),2);
data3 = decode_32bit(data(1616:1619),2);
data4 = decode_32bit(data(1620:1623),2);
data5 = decode_32bit(data(1624:1627),2);
tcp_queue_level = decode_32bit(data(1628:1631),1);
fifo_queue_level = decode_32bit(data(1632:1635),1);

% games
double_tap_counter = decode_32bit(data(1640:1643),1);
finish_line_counter = decode_32bit(data(1644:1647),1);

% pressure_raw
up = decode_32bit(data(1652:1655),2);
ut = decode_16bit(data(1656:1657),1);
Temperature_meas = decode_32bit(data(1658:1661),2);
Precission_meas = decode_32bit(data(1662:1665),2);

% magneto
mx = decode_16bit(data(1670:1671),1);
my = decode_16bit(data(1672:1673),1);
mz = decode_16bit(data(1674:1675),1);
magneto_raw(1) = decode_32bit(data(1676:1679),0);
magneto_raw(2) = decode_32bit(data(1680:1683),0);
magneto_raw(3) = decode_32bit(data(1684:1687),0);
magneto_rectified(1) = decode_32bit(data(1688:1691),0);
magneto_rectified(2) = decode_32bit(data(1692:1695),0);
magneto_rectified(3) = decode_32bit(data(1696:1699),0);
magneto_offset(1) = decode_32bit(data(1700:1703),0);
magneto_offset(2) = decode_32bit(data(1704:1707),0);
magneto_offset(3) = decode_32bit(data(1708:1711),0);
heading_unwrapped = decode_32bit(data(1712:1715),0);
heading_gyro_unwrapped = decode_32bit(data(1716:1719),0);
heading_fusion_unwrapped = decode_32bit(data(1720:1723),0);
magneto_calibration_ok = char(data(1724:1732));
magneto_state = decode_32bit(data(1733:1736),1);
magneto_radius = decode_32bit(data(1737:1740),0);
error_mean = decode_32bit(data(1741:1744),0);
error_var = decode_32bit(data(1745:1748),0);

% wind speed
wind_speed = decode_32bit(data(1753:1756),0);
wind_angle = decode_32bit(data(1757:1760),0);
wind_compensation_theta = decode_32bit(data(1761:1764),0);
wind_compensation_phi = decode_32bit(data(1765:1768),0);
state_x1 = decode_32bit(data(1769:1772),0);
state_x2 = decode_32bit(data(1773:1776),0);
state_x3 = decode_32bit(data(1777:1780),0);
state_x4 = decode_32bit(data(1781:1784),0);
state_x5 = decode_32bit(data(1785:1788),0);
state_x6 = decode_32bit(data(1789:1792),0);
magneto_debug1 = decode_32bit(data(1793:1796),0);
magneto_debug2 = decode_32bit(data(1797:1800),0);
magneto_debug3 = decode_32bit(data(1801:1804),0);
% 8 bytes unacounted for!!

% kalman pressure
offset_pressure = decode_32bit(data(1817:1820),0);
est_z = decode_32bit(data(1821:1824),0);
est_zdot = decode_32bit(data(1825:1828),0);
est_bias_PWM = decode_32bit(data(1829:1832),0);
est_biais_pression = decode_32bit(data(1833:1836),0);
offset_US = decode_32bit(data(1837:1840),0);
prediction_US = decode_32bit(data(1841:1844),0);
cov_alt = decode_32bit(data(1817:1848),0);
cov_PWM = decode_32bit(data(1849:1852),0);
cov_vitesse = decode_32bit(data(1853:1856),0);
bool_effect_sol = data(1857);
somme_inno = decode_32bit(data(1861:1864),0);
flag_reject_US = data(1865);
u_multisinus = decode_32bit(data(1869:1872),0);
gaz_altitude = decode_32bit(data(1873:1876),0);
Flag_multissinus = data(1877);
Flag_multissinus_debut = data(1881);

% hdvideo stream
hdvideo_state = decode_32bit(data(1889:1892),1);
storage_fifo_nb_packets = decode_32bit(data(1893:1896),1);
storage_fifo_size = decode_32bit(data(1897:1900),1);
usbkey_size = decode_32bit(data(1901:1904),1);
usbkey_freespace = decode_32bit(data(1905:1908),1);
hdframe_number = decode_32bit(data(1909:1912),1);
usbkey_reamining_time = decode_32bit(data(1913:1916),1);

% wifi
link_quality = decode_32bit(data(1921:1924),1);

% zimmu_3000 - deprecated

%cks
cks = decode_32bit(data(end-3:end),1);

if (ardrone_state(32) ==1 && altitude< 0.2   )
    altitude = hPrev;
elseif ardrone_state(32)==1 
    hPrev= altitude; 
end
  
    
end


function res = decode_32bit(input, mark)
% if mark = 1; then output a int
% else output the float value which is defined by SDK description.
% the input is an array (1*4)
% e.g. : NDS(Battery_OS:Battery_OS+data_length-1)
hex_value = dec2hex(input);
hex_value = [hex_value(4,:),hex_value(3,:),hex_value(2,:),hex_value(1,:)];
if mark ==1
    res = hex2dec(hex_value);
elseif mark ==2
    res = hex2dec(hex_value)-2^31;
else
    res = typecast(uint32(hex2dec(hex_value)),'single');
end
end

function res = decode_16bit(input,mark)
hex_value = dec2hex(input);
hex_value = [hex_value(2,:),hex_value(1,:)];
res = hex2dec(hex_value);
if mark==1
    res=res-2^15;
end
end

function bin = getDroneState(input)
bin = zeros(32,1);
hex = dec2hex(input);
% put the hex_value in the order [31, 30......0]
hex = [hex(4,:),hex(3,:),hex(2,:),hex(1,:)];
for i=1:length(hex)
    if hex(i)=='F'
        bin((i*4)-3:i*4)=[1 1 1 1];
    elseif hex(i)=='E'
        bin((i*4)-3:i*4)=[1 1 1 0];
    elseif hex(i)=='D'
        bin((i*4)-3:i*4)=[1 1 0 1];
    elseif hex(i)=='C'
        bin((i*4)-3:i*4)=[1 1 0 0];
    elseif hex(i)=='B'
        bin((i*4)-3:i*4)=[1 0 1 1];
    elseif hex(i)=='A'
        bin((i*4)-3:i*4)=[1 0 1 0];
    elseif hex(i)=='9'
        bin((i*4)-3:i*4)=[1 0 0 1];
    elseif hex(i)=='8'
        bin((i*4)-3:i*4)=[1 0 0 0];
    elseif hex(i)=='7'
        bin((i*4)-3:i*4)=[0 1 1 1];
    elseif hex(i)=='6'
        bin((i*4)-3:i*4)=[0 1 1 0];
    elseif hex(i)=='5'
        bin((i*4)-3:i*4)=[0 1 0 1];
    elseif hex(i)=='4'
        bin((i*4)-3:i*4)=[0 1 0 0];
    elseif hex(i)=='3'
        bin((i*4)-3:i*4)=[0 0 1 1];
    elseif hex(i)=='2'
        bin((i*4)-3:i*4)=[0 0 1 0];
    elseif hex(i)=='1'
        bin((i*4)-3:i*4)=[0 0 0 1];
    elseif hex(i)=='0'
        bin((i*4)-3:i*4)=[0 0 0 0];
    end
end

end

== matlab function ARDroneHover_AMOSTROU/ARDrone Wi-Fi  Block/Data synchronization  ==
  data: dataIn input; frameOut output; flagOut output
function [frameOut,flagOut]  = fcn(dataIn)
%#eml
%% Author: David Escobar Sanabria
%  Description: This function synchronizes data coming from the flight computer
%  computer. 
%  frameOut: Organized frame
%  frameIn: sequence of bytes not sync.
persistent frame; 
persistent lastFrame; 
persistent count; 
persistent countHeader; 
persistent countBuffer; 
persistent buffer; 

%% Size of byte array containing the data
sizePayload= 2186;

%% Size of the array read each time step
nBytes = 2190 ;%size(dataIn,1); 


%%%%%%%%%%%%%%%%%%%%%%%%%%%%%%%%%%%%%%%%%%%%%%%%%%%%%%%
%% Initialization of presistent variables
if isempty(buffer)
    buffer=uint8(zeros(10000,1));
end

if isempty(countBuffer)
    countBuffer=0;
end


if isempty(frame)
    frame=uint8(zeros(sizePayload,1));
end

if isempty(lastFrame)
    lastFrame=uint8(zeros(sizePayload,1));
end


if isempty(count)
    count=0;
end

if isempty(countHeader)
    countHeader=0;
end
%%%%%%%%%%%%%%%%%%%%%%%%%%%%%%%%%%%%%%%%%%%%%%%%%%%%%%%

%% Filling the buffer
buffer(countBuffer+1:countBuffer+nBytes) = dataIn;

bytesToRead = countBuffer+nBytes; 

%%%%%%%%%%%%%%%%%%%%%%%%%%%%%%%%%%%%%%%%%%%%%%%%%%%%%%%
%% Reading buffer

for k=1:bytesToRead    
    if(countHeader==4 && count<sizePayload)
        bytesLeft = sizePayload-count;
        frame(count+1:sizePayload) = buffer(k:k+bytesLeft-1);
        count = sizePayload;
        countBuffer = bytesToRead-bytesLeft ;
        buffer(1:countBuffer) = buffer(k+bytesLeft:bytesToRead);
        break;
        
    end
    
    if(countHeader==3 && buffer(k)==85)
        
        countHeader=4;
 
        if(bytesToRead-k > sizePayload)
            count =sizePayload;  
            frame(1:count) = buffer(k+1:k+sizePayload);  
            countBuffer =bytesToRead-k-sizePayload ; 
            buffer(1:countBuffer) = buffer(k+sizePayload+1:bytesToRead);
        else
            
            count =bytesToRead-k;
            if count > 0          
                frame(1:count) = buffer(k+1:bytesToRead);  
            end
            countBuffer = 0; 
            
        end
        
        break;
    end
    
    if(countHeader==2 && buffer(k)==102)
        countHeader=3;
    end
    
    if(countHeader==1 && buffer(k)==119)
        countHeader=2;
    end
       
    if(countHeader==0 && buffer(k)==136)
        countHeader=1;
    end

end

if count==sizePayload 
     frameOut = frame(1:sizePayload,1); % forcei tamanho maximo...
     flagOut = 1; 
     lastFrame = frame;
     frame=uint8(zeros(sizePayload,1));
     count=0;
     countHeader=0;
     
else % In case the buffer does not have an entire payload
    frameOut = lastFrame;
    flagOut = 0; 
end

== matlab function ARDroneHover_AMOSTROU/ARDrone Wi-Fi  Block/Subsystem1/Drone state request ==
  data: status input; fly input; rollAngRef input; pitchAngRef input; yawRateRef input; wRef input; enableRefs input; dataControl output; isFlying output; stop input; error output
function [dataControl, isFlying, error] = fcn( status, fly, rollAngRef, pitchAngRef, yawRateRef, wRef, enableRefs, stop)
%#codegen

% Persistent variables.
persistent SequenceNumber ;

% Initialization of persistent variables at first time step. 

if isempty(SequenceNumber)
    SequenceNumber = 1 ;
end



% Error code / No error: 0
error=0;

% Boolean of flying status / Flying: 1
isFlying = status(32) ;

% Byte array of size 150 to be sent to the drone.
strOut = uint8(zeros(150,1)) ;

% String that coontains a variable size command. 
% cmd is concatenated with previous commands at each sample
cmd = '';

% At first time step and every 100 time steps, data is requested.
if (SequenceNumber <=1 || mod(SequenceNumber, 100) ==0 )
    SequenceNumber = SequenceNumber+1; 
    strCmd = getString(SequenceNumber) ;
    cmd = ['AT*CONFIG=' strCmd ',"general:navdata_demo","FALSE"' char(13)];
    
end

SequenceNumber = SequenceNumber+1;
strCmd = getString(SequenceNumber) ;
cmd = [cmd 'AT*COMWDG=' strCmd char(13)];


if stop ==1 % Emergency stop
   cmd = ['AT*REF=' strCmd ',290717952' char(13)] ; 
    
else % Not emergency stop
    
    if SequenceNumber >20 && SequenceNumber <22
        
        % Trim vehicle state estimation / angles set to zero
        SequenceNumber =SequenceNumber+1;
        strCmd = getString(SequenceNumber) ;
        cmd = [cmd 'AT*FTRIM=' strCmd char(13)] ;
        
    elseif SequenceNumber >=22 && SequenceNumber <25
        cmd = [cmd 'AT*CONFIG=' strCmd '"conrol:altitude_max","100000"' char(13)] ;
        
        
    elseif SequenceNumber >=25
        
        if ( fly == 1  )
            
            if (isFlying ==0)
                
                SequenceNumber =SequenceNumber+1;
                strCmd = getString(SequenceNumber) ;
                cmd = [cmd 'AT*REF=' strCmd ',290718208' char(13)] ;
                
            elseif isFlying==1 && enableRefs==1
                
                SequenceNumber =SequenceNumber+1;
                strCmd = getString(SequenceNumber) ;
                      
                cmd = [cmd 'AT*PCMD=' strCmd ',1,'] ;
                 
                aux = double (float2IEEE754 (rollAngRef) )  ;
                strAux = getString(abs(aux)) ; 
                if rollAngRef<0
                   strAux = [char(45) strAux] ; 
                end
                cmd = [cmd strAux ','];
                      
               aux = double (float2IEEE754 (pitchAngRef) ) ;
               strAux = getString(abs(aux)) ; 
               if pitchAngRef<0
                    strAux = [char(45) strAux] ; 
               end
               cmd = [cmd strAux ','];
                      
               aux =  double(float2IEEE754 (wRef)) ;
               strAux = getString(abs(aux)) ; 
               if wRef<0
                    strAux = [char(45) strAux] ; 
               end
               cmd = [cmd strAux ','];
                      
                      
               aux =  double (float2IEEE754 (yawRateRef) ) ;
               strAux = getString(abs(aux)) ; 
               if yawRateRef <0
                     error=2; 
                     strAux = [char(45) strAux] ; 
               end
               cmd = [cmd strAux char(13)];
               
                
            end
            
            
        elseif ( fly==0 )
                
               if isFlying ==1
                    SequenceNumber =SequenceNumber+1;
                    strCmd = getString(SequenceNumber) ;
                    cmd = [cmd 'AT*REF=' strCmd ',290717696' char(13)] ;
                    
               end
        end
        
    end
    
%     SequenceNumber =SequenceNumber+1;
%     strCmd = getString(SequenceNumber) ;
%     cmd = [cmd 'AT*PWM=' strCmd ',0,0,0,0'] ;
    
end

% cmd must contain less than 150 bytes. 
if (length(cmd)<150)
    strOut(1:length(cmd)) = cmd ;
else
    error =1; 
end

dataControl = strOut;

end


%% My str2num function that allows for code generation
function [ strOut] = getString( a )
d=1;

if (a<10)
    d=1;
end

if (a >=10 && a <100)
    d=2;
end

if (a >=100 && a <1000)
    d=3;
end

if (a >=1000 && a <10000)
    d=4;
end

if (a >=10000 && a <100000)
    d=5;
end

if (a >=100000 && a <1000000)
    d=6;
end

if (a >=1000000 && a <10000000)
    d=7;
end

if (a >=10000000 && a <100000000)
    d=8;
end

if (a >=100000000 && a <1000000000)
    d=9;
end

if (a >=1000000000 && a <10000000000)
    d=10;
end

if (a >=10000000000 )
    d=11;
end



digit = uint8(zeros(1,d)) ;
resTotal = 0;
%d = length(a) ;
for k=1:d
    
    res1 = mod(a,10^k)/(10^(k-1)) ;
    %( mod(a,10*k) - resTotal)/(10*k) ;
    
    digit(d-k+1) = char(48 + res1);
    resTotal = (10^(k-1))*res1 +resTotal;
    
end

strOut = char(digit) ;


end

%% Function to obtain a IEEE754 representation of a float number
function [ iVal ] = float2IEEE754( fVal )

binData = dec2bin(typecast (single(fVal), 'uint8'),8) ;

binData2 =[ binData(4,:) binData(3,:) binData(2,:) binData(1,:)] ;
iVal =0; 
for k=32:-1:1
    
    if (binData2(k) =='1')
        bit = 1;
    else
        bit =0;
    end
    
    if k == 1
        iVal = iVal - bit*2^(31);
    else
        iVal = iVal + bit*2^(32-k) ; 
    end
    
end

iVal = int32(iVal);

end
